simulink model "EKM_SL"  (R2018b)
settings: Solver=VariableStepAuto  StartTime=0.0  StopTime=10.0  RelTol=1e-3
undefined symbols (not defined in the file or in its folder): EKM
libraries: simulink x1
settings Model: Creator=Szalay  LastModifiedBy=Szalay

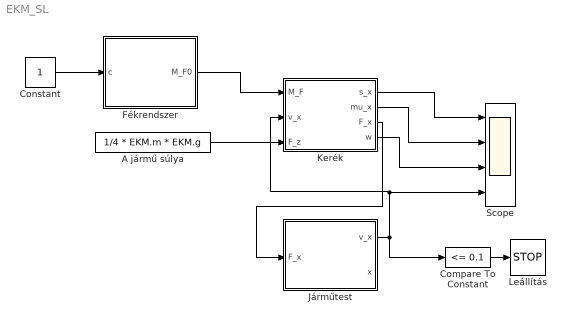
== system EKM_SL ==
  A jármű súlya : Constant  Value=1/4 * EKM.m * EKM.g
  Compare To Constant : simulink/Logic and Bit Operations/Compare To Constant  relop=<=  const=0.1  OutDataTypeStr=boolean
  Constant : Constant
  Fékrendszer : Subsystem  mask(Fékmodell){V_0=EKM.V_0, T_D=EKM.T_D, C_q=EKM.C_q, p_0=EKM.p_0, A_F=EKM.A_F, mu_F=EKM.mu_F, R_F=EKM.R_F}
      mask prompts: V_0 "Haszontalan térfogat"; T_D "Fékholtidő"; C_q "Összevont fékjellemző"; p_0 "A főfékhenger nyomása [kPa]"; A_F "A fékmunkahenger keresztmetszete"; mu_F "Féksúrlódási együttható"; R_F "A féktárcsa közepes sugara"
      mask help: Hidraulikus fékmodell.
      mask DialogControl ParameterGroupVar Prompt: Hidraulikus fékmodell
      mask DialogControl Container3 Prompt: Tárcsa és pofák
  Járműtest : Subsystem  mask(Járműtest){m=EKM.m, c_W=EKM.c_W, rho_L=EKM.rho, A_0=EKM.A, v_0=10, x_0=0}
      mask prompts: m "Tömeg"; c_W "Légellenellási tényező"; rho_L "A levegő sűrűsége"; A_0 "Homlokfelület"; v_0 "Kezdeti sebesség"; x_0 "Kezdeti hely"
      mask help: Járműtest negyed tömeggel és légellenállással.
      mask DialogControl ParameterGroupVar Prompt: A járműtest tömege
      mask DialogControl Container3 Prompt: Légellenállás
      mask DialogControl Container4 Prompt: Kezdeti értékek
  Kerék : Subsystem  mask(Kerékmodell){R=EKM.R, J=EKM.J, B=EKM.B, w_0=10/EKM.R}
      mask prompts: R "Keréksugár"; J "Tehetetlenségi nyomaték"; B "Forgási súrlódási tényező"; w_0 "Kezdeti szögsebesség"
      mask help: A kerékmodell Pacejka-féle gumiabroncsmodellel és féknyomaték-korlátozással.
      mask DialogControl ParameterGroupVar Prompt: Kerékjellemzők
      mask DialogControl Container3 Prompt: Hajtáslánc jellemzők
      mask DialogControl Container4 Prompt: Kezdeti értékek
  Leállítás : Stop
  Scope : Scope  NumInputPorts=4
  wires:
  Járműtest/1(v_x) -> Compare To Constant/1, Kerék/2(v_x), Scope/4
  Kerék/3(F_x) -> Járműtest/1(F_x)
  A jármű súlya/1 -> Kerék/3(F_z)
  Kerék/1(s_x) -> Scope/1
  Kerék/2(mu_x) -> Scope/2
  Kerék/4(w) -> Scope/3
  Compare To Constant/1 -> Leállítás/1
  Fékrendszer/1(M_F0) -> Kerék/1(M_F)
  Constant/1 -> Fékrendszer/1(c)

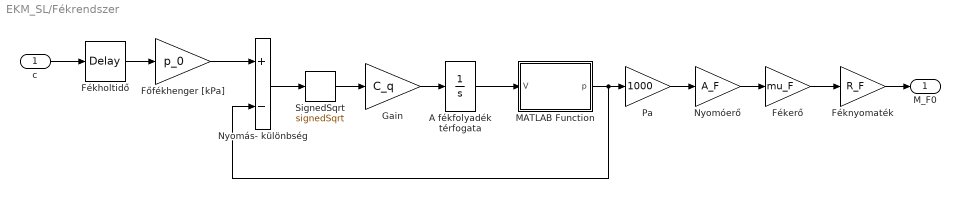
== system EKM_SL/Fékrendszer ==
  c : Inport
  A fékfolyadék térfogata : Integrator  LimitOutput=on  LowerSaturationLimit=0
  Fékerő : Gain  Gain=mu_F
  Fékholtidő : TransportDelay  DelayTime=T_D
  Féknyomaték : Gain  Gain=R_F
  Főfékhenger [kPa] : Gain  Gain=p_0
  Gain : Gain  Gain=C_q
  MATLAB Function : MATLAB Function  TreatAsAtomicUnit=on
  Nyomás- különbség : Sum  Inputs=+-
  Nyomóerő : Gain  Gain=A_F
  Pa : Gain  Gain=1000
  SignedSqrt : Sqrt  Operator=signedSqrt  IntermediateResultsDataTypeStr=single  SaturateOnIntegerOverflow=on
  M_F0 : Outport
  wires:
  Nyomás- különbség/1 -> SignedSqrt/1
  SignedSqrt/1 -> Gain/1
  Gain/1 -> A fékfolyadék térfogata/1
  Főfékhenger [kPa]/1 -> Nyomás- különbség/1
  c/1 -> Fékholtidő/1
  Fékholtidő/1 -> Főfékhenger [kPa]/1
  A fékfolyadék térfogata/1 -> MATLAB Function/1(V)
  MATLAB Function/1(p) -> Nyomás- különbség/2, Pa/1
  Pa/1 -> Nyomóerő/1
  Nyomóerő/1 -> Fékerő/1
  Féknyomaték/1 -> M_F0/1
  Fékerő/1 -> Féknyomaték/1

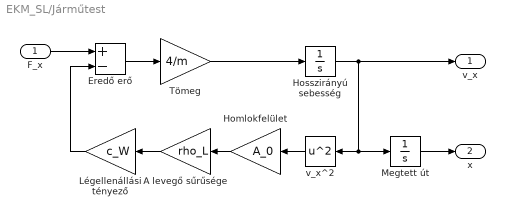
== system EKM_SL/Járműtest ==
  F_x : Inport
  A levegő sűrűsége : Gain  Gain=rho_L
  Eredő erő : Sum  Inputs=+-
  Homlokfelület : Gain  Gain=A_0
  Hosszirányú sebesség : Integrator  InitialCondition=v_0
  Légellenállási tényező : Gain  Gain=c_W
  Megtett út : Integrator  InitialCondition=x_0
  Tömeg : Gain  Gain=4/m
  v_x^2 : Math  Operator=square  SaturateOnIntegerOverflow=on
  v_x : Outport
  x : Outport  Port=2
  wires:
  Tömeg/1 -> Hosszirányú sebesség/1
  Hosszirányú sebesség/1 -> v_x/1, v_x^2/1, Megtett út/1
  Eredő erő/1 -> Tömeg/1
  F_x/1 -> Eredő erő/1
  Megtett út/1 -> x/1
  v_x^2/1 -> Homlokfelület/1
  Homlokfelület/1 -> A levegő sűrűsége/1
  A levegő sűrűsége/1 -> Légellenállási tényező/1
  Légellenállási tényező/1 -> Eredő erő/2

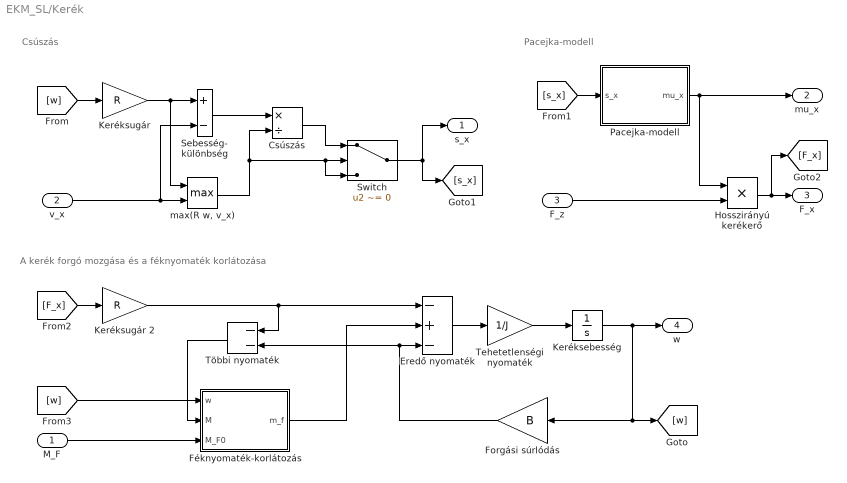
== system EKM_SL/Kerék ==
  note: A kerék forgó mozgása és a féknyomaték korlátozása
  note: Pacejka-modell
  note: Csúszás
  M_F : Inport
  v_x : Inport  Port=2
  F_z : Inport  Port=3
  Csúszás : Product  Inputs=*/
  Eredő nyomaték : Sum  Inputs=-+-
  Forgási súrlódás : Gain  Gain=B
  Féknyomaték-korlátozás : MATLAB Function  TreatAsAtomicUnit=on
  Hosszirányú kerékerő : Product
  Keréksebesség : Integrator  InitialCondition=w_0
  Keréksugár : Gain  Gain=R
  Keréksugár 2 : Gain  Gain=R
  Pacejka-modell : MATLAB Function  TreatAsAtomicUnit=on
  Sebesség- különbség : Sum  Inputs=+-
  Switch : Switch  Criteria=u2 ~= 0
  Tehetetlenségi nyomaték : Gain  Gain=1/J
  Többi nyomaték : Sum  Inputs=--
  "max(R w, v_x)" : MinMax  Function=max  Inputs=2
  s_x : Outport
  mu_x : Outport  Port=2
  F_x : Outport  Port=3
  w : Outport  Port=4
  wires:
  Eredő nyomaték/1 -> Tehetetlenségi nyomaték/1
  Forgási súrlódás/1 -> Többi nyomaték/2, Eredő nyomaték/3
  Keréksebesség/1 -> w/1, [w], Forgási súrlódás/1
  Tehetetlenségi nyomaték/1 -> Keréksebesség/1
  [w] -> Keréksugár/1
  Keréksugár/1 -> "max(R w, v_x)"/1, Sebesség- különbség/1
  v_x/1 -> "max(R w, v_x)"/2, Sebesség- különbség/2
  Sebesség- különbség/1 -> Csúszás/1
  "max(R w, v_x)"/1 -> Switch/3, Switch/2, Csúszás/2
  [s_x] -> Pacejka-modell/1(s_x)
  Pacejka-modell/1(mu_x) -> mu_x/1, Hosszirányú kerékerő/1
  F_z/1 -> Hosszirányú kerékerő/2
  Hosszirányú kerékerő/1 -> [F_x], F_x/1
  [F_x] -> Keréksugár 2/1
  Keréksugár 2/1 -> Többi nyomaték/1, Eredő nyomaték/1
  M_F/1 -> Féknyomaték-korlátozás/3(M_F0)
  Többi nyomaték/1 -> Féknyomaték-korlátozás/2(M)
  [w] -> Féknyomaték-korlátozás/1(w)
  Féknyomaték-korlátozás/1(m_f) -> Eredő nyomaték/2
  Switch/1 -> s_x/1, [s_x]
  Csúszás/1 -> Switch/1

== matlab function EKM_SL/Kerék/Pacejka-modell ==
  data: s_x input; mu_x output
function mu_x = Pacejka(s_x)

mu_x = EKM.Pacejka(s_x);

== matlab function EKM_SL/Fékrendszer/MATLAB Function ==
  data: V input; p output
function p = F(V)

p = EKM.BrakeModel(V);

== matlab function EKM_SL/Kerék/Féknyomaték-korlátozás ==
  data: w input; m_f output; M input; M_F0 input
function m_f = M_F(w, M, M_F0)

m_f = EKM.M_F(w, M, M_F0);
